simulink model "rls_est"  (R2017b)
settings: Solver=FixedStepAuto  StartTime=0.0  StopTime=tEnd  FixedStep=dt  RelTol=1e-3
values from neighbouring files (symbols this model uses):
  dt = t(2)-t(1)    [greybox_sys_id.m]    (also in kalman_filter.m; ls_regression.m; rls_estimation.m; sys_id.m)
libraries: ctrlSharedLib x8
settings Model: Creator=e_anderlini  LastModifiedBy=e_anderlini
settings CodeAppCC: StateflowObjectComments=on

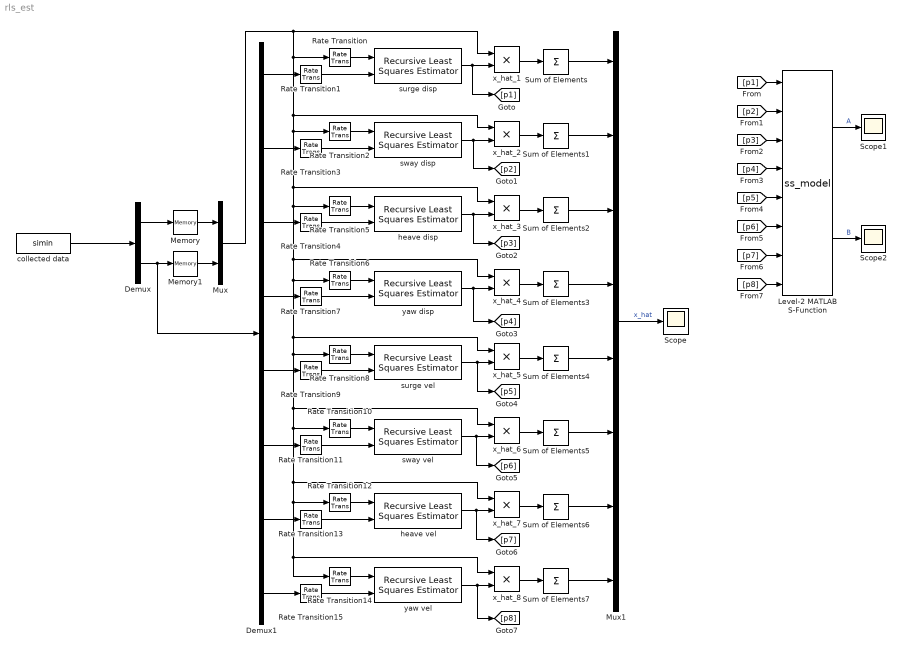
== system rls_est ==
  Demux : Demux  Outputs=[4,8]
  Demux1 : Demux  Outputs=8
  Level-2 MATLAB S-Function : M-S-Function  FunctionName=ss_model
  Memory : Memory
  Memory1 : Memory
  Mux : Mux  Inputs=2
  Mux1 : Mux  Inputs=8
  Rate Transition{,1..15} (16 alike) : RateTransition  OutPortSampleTime=dt
  Scope : Scope
  Scope1 : Scope
  Scope2 : Scope
  Sum of Elements{,1..7} (8 alike) : Sum  Inputs=+
  collected data : FromWorkspace  VariableName=simin  SampleTime=0
  heave disp : ctrlSharedLib/Recursive Least Squares Estimator  InitialEstimateSource=None  InitialParameterData=12  P0=R  EstimationMethod=Forgetting Factor  AdaptationParameter=0.99  HasTimeVaryingAdaptationParameter=off  NormalizationBias=eps  OutputError=off  OutputP=off  AddEnablePort=off  Ts=dt
      settings: SourceProductName=Control System Toolbox  SourceProductBaseCode=CT
  heave vel : ctrlSharedLib/Recursive Least Squares Estimator  InitialEstimateSource=None  InitialParameterData=12  P0=R  EstimationMethod=Forgetting Factor  AdaptationParameter=0.99  HasTimeVaryingAdaptationParameter=off  NormalizationBias=eps  OutputError=off  OutputP=off  AddEnablePort=off  Ts=dt
      settings: SourceProductName=Control System Toolbox  SourceProductBaseCode=CT
  surge disp : ctrlSharedLib/Recursive Least Squares Estimator  InitialEstimateSource=None  InitialParameterData=12  P0=R  EstimationMethod=Forgetting Factor  AdaptationParameter=0.99  HasTimeVaryingAdaptationParameter=off  NormalizationBias=eps  OutputError=off  OutputP=off  AddEnablePort=off  Ts=dt
      settings: SourceProductName=Control System Toolbox  SourceProductBaseCode=CT
  surge vel : ctrlSharedLib/Recursive Least Squares Estimator  InitialEstimateSource=None  InitialParameterData=12  P0=R  EstimationMethod=Forgetting Factor  AdaptationParameter=0.99  HasTimeVaryingAdaptationParameter=off  NormalizationBias=eps  OutputError=off  OutputP=off  AddEnablePort=off  Ts=dt
      settings: SourceProductName=Control System Toolbox  SourceProductBaseCode=CT
  sway disp : ctrlSharedLib/Recursive Least Squares Estimator  InitialEstimateSource=None  InitialParameterData=12  P0=R  EstimationMethod=Forgetting Factor  AdaptationParameter=0.99  HasTimeVaryingAdaptationParameter=off  NormalizationBias=eps  OutputError=off  OutputP=off  AddEnablePort=off  Ts=dt
      settings: SourceProductName=Control System Toolbox  SourceProductBaseCode=CT
  sway vel : ctrlSharedLib/Recursive Least Squares Estimator  InitialEstimateSource=None  InitialParameterData=12  P0=R  EstimationMethod=Forgetting Factor  AdaptationParameter=0.99  HasTimeVaryingAdaptationParameter=off  NormalizationBias=eps  OutputError=off  OutputP=off  AddEnablePort=off  Ts=dt
      settings: SourceProductName=Control System Toolbox  SourceProductBaseCode=CT
  x_hat_{1..8} (8 alike) : Product
  yaw disp : ctrlSharedLib/Recursive Least Squares Estimator  InitialEstimateSource=None  InitialParameterData=12  P0=R  EstimationMethod=Forgetting Factor  AdaptationParameter=0.99  HasTimeVaryingAdaptationParameter=off  NormalizationBias=eps  OutputError=off  OutputP=off  AddEnablePort=off  Ts=dt
      settings: SourceProductName=Control System Toolbox  SourceProductBaseCode=CT
  yaw vel : ctrlSharedLib/Recursive Least Squares Estimator  InitialEstimateSource=None  InitialParameterData=12  P0=R  EstimationMethod=Forgetting Factor  AdaptationParameter=0.99  HasTimeVaryingAdaptationParameter=off  NormalizationBias=eps  OutputError=off  OutputP=off  AddEnablePort=off  Ts=dt
      settings: SourceProductName=Control System Toolbox  SourceProductBaseCode=CT
  wires:
  Mux1/1 -> Scope/1  "x_hat"
  Demux/1 -> Memory/1
  Memory1/1 -> Mux/2
  Memory/1 -> Mux/1
  surge disp/1 -> [p1], x_hat_1/2
  yaw vel/1 -> [p8], x_hat_8/2
  sway disp/1 -> [p2], x_hat_2/2
  heave disp/1 -> [p3], x_hat_3/2
  yaw disp/1 -> [p4], x_hat_4/2
  surge vel/1 -> [p5], x_hat_5/2
  sway vel/1 -> [p6], x_hat_6/2
  heave vel/1 -> [p7], x_hat_7/2
  x_hat_1/1 -> Sum of Elements/1
  x_hat_2/1 -> Sum of Elements1/1
  x_hat_3/1 -> Sum of Elements2/1
  x_hat_4/1 -> Sum of Elements3/1
  x_hat_5/1 -> Sum of Elements4/1
  x_hat_6/1 -> Sum of Elements5/1
  x_hat_7/1 -> Sum of Elements6/1
  x_hat_8/1 -> Sum of Elements7/1
  Sum of Elements/1 -> Mux1/1
  Sum of Elements1/1 -> Mux1/2
  Sum of Elements2/1 -> Mux1/3
  Sum of Elements3/1 -> Mux1/4
  Sum of Elements4/1 -> Mux1/5
  Sum of Elements5/1 -> Mux1/6
  Sum of Elements6/1 -> Mux1/7
  Sum of Elements7/1 -> Mux1/8
  Demux1/1 -> Rate Transition1/1
  Demux1/2 -> Rate Transition3/1
  Demux1/3 -> Rate Transition4/1
  Demux1/4 -> Rate Transition7/1
  Demux1/5 -> Rate Transition9/1
  Demux1/6 -> Rate Transition11/1
  Demux1/7 -> Rate Transition13/1
  Demux1/8 -> Rate Transition15/1
  Demux/2 -> Demux1/1, Memory1/1
  collected data/1 -> Demux/1
  Rate Transition/1 -> surge disp/1
  Rate Transition1/1 -> surge disp/2
  Mux/1 -> x_hat_1/1, Rate Transition/1, x_hat_2/1, Rate Transition2/1, x_hat_3/1, Rate Transition5/1, x_hat_4/1, Rate Transition6/1, x_hat_5/1, Rate Transition8/1, x_hat_6/1, Rate Transition10/1, x_hat_7/1, Rate Transition12/1, x_hat_8/1, Rate Transition14/1
  Rate Transition3/1 -> sway disp/2
  Rate Transition2/1 -> sway disp/1
  Rate Transition4/1 -> heave disp/2
  Rate Transition5/1 -> heave disp/1
  Rate Transition6/1 -> yaw disp/1
  Rate Transition7/1 -> yaw disp/2
  Rate Transition8/1 -> surge vel/1
  Rate Transition9/1 -> surge vel/2
  Rate Transition10/1 -> sway vel/1
  Rate Transition11/1 -> sway vel/2
  Rate Transition12/1 -> heave vel/1
  Rate Transition13/1 -> heave vel/2
  Rate Transition14/1 -> yaw vel/1
  Rate Transition15/1 -> yaw vel/2
  Level-2 MATLAB S-Function/2 -> Scope2/1  "B"
  Level-2 MATLAB S-Function/1 -> Scope1/1  "A"
  [p1] -> Level-2 MATLAB S-Function/1
  [p2] -> Level-2 MATLAB S-Function/2
  [p3] -> Level-2 MATLAB S-Function/3
  [p4] -> Level-2 MATLAB S-Function/4
  [p5] -> Level-2 MATLAB S-Function/5
  [p6] -> Level-2 MATLAB S-Function/6
  [p7] -> Level-2 MATLAB S-Function/7
  [p8] -> Level-2 MATLAB S-Function/8
